simulink model "mainModelDOEJF"  (R2025a)
settings: Solver=VariableStepAuto  StartTime=0  StopTime=1000  RelTol=1e-3
undefined symbols (not defined in the file): advectiveCoefficientScale, AmbientTemperature, coolantTempSourceTemperatureScale, massCoolantScale, massModuleScale, scaledAdvectiveCoefficient, scaledCoolantTemp, scaledMassCoolant, scaledMassModule
libraries: fl_lib x265, nesl_utility x68, coolantFlow_lib x65, thermalCoupledCellResolution_lib x32, heatGenerationForCellResolvedModel x32, batt_lib x1, coolantFlowSwitch_lib x1
(part 2 of 4)

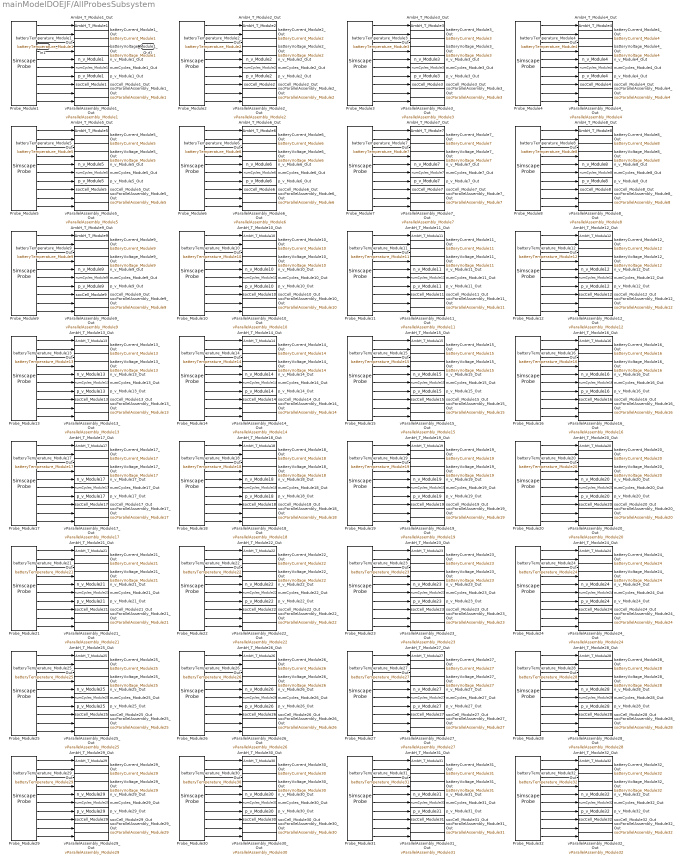
== system mainModelDOEJF/AllProbesSubsystem ==
  In1 : Inport
  AmbH_T_Module10_Out : ToWorkspace  VariableName=AmbH_T_Module10  SaveFormat=Structure With Time  SampleTime=-1
  AmbH_T_Module11_Out : ToWorkspace  VariableName=AmbH_T_Module11  SaveFormat=Structure With Time  SampleTime=-1
  AmbH_T_Module12_Out : ToWorkspace  VariableName=AmbH_T_Module12  SaveFormat=Structure With Time  SampleTime=-1
  AmbH_T_Module13_Out : ToWorkspace  VariableName=AmbH_T_Module13  SaveFormat=Structure With Time  SampleTime=-1
  AmbH_T_Module14_Out : ToWorkspace  VariableName=AmbH_T_Module14  SaveFormat=Structure With Time  SampleTime=-1
  AmbH_T_Module15_Out : ToWorkspace  VariableName=AmbH_T_Module15  SaveFormat=Structure With Time  SampleTime=-1
  AmbH_T_Module16_Out : ToWorkspace  VariableName=AmbH_T_Module16  SaveFormat=Structure With Time  SampleTime=-1
  AmbH_T_Module17_Out : ToWorkspace  VariableName=AmbH_T_Module17  SaveFormat=Structure With Time  SampleTime=-1
  AmbH_T_Module18_Out : ToWorkspace  VariableName=AmbH_T_Module18  SaveFormat=Structure With Time  SampleTime=-1
  AmbH_T_Module19_Out : ToWorkspace  VariableName=AmbH_T_Module19  SaveFormat=Structure With Time  SampleTime=-1
  AmbH_T_Module1_Out : ToWorkspace  VariableName=AmbH_T_Module1  SaveFormat=Structure With Time  SampleTime=-1
  AmbH_T_Module20_Out : ToWorkspace  VariableName=AmbH_T_Module20  SaveFormat=Structure With Time  SampleTime=-1
  AmbH_T_Module21_Out : ToWorkspace  VariableName=AmbH_T_Module21  SaveFormat=Structure With Time  SampleTime=-1
  AmbH_T_Module22_Out : ToWorkspace  VariableName=AmbH_T_Module22  SaveFormat=Structure With Time  SampleTime=-1
  AmbH_T_Module23_Out : ToWorkspace  VariableName=AmbH_T_Module23  SaveFormat=Structure With Time  SampleTime=-1
  AmbH_T_Module24_Out : ToWorkspace  VariableName=AmbH_T_Module24  SaveFormat=Structure With Time  SampleTime=-1
  AmbH_T_Module25_Out : ToWorkspace  VariableName=AmbH_T_Module25  SaveFormat=Structure With Time  SampleTime=-1
  AmbH_T_Module26_Out : ToWorkspace  VariableName=AmbH_T_Module26  SaveFormat=Structure With Time  SampleTime=-1
  AmbH_T_Module27_Out : ToWorkspace  VariableName=AmbH_T_Module27  SaveFormat=Structure With Time  SampleTime=-1
  AmbH_T_Module28_Out : ToWorkspace  VariableName=AmbH_T_Module28  SaveFormat=Structure With Time  SampleTime=-1
  AmbH_T_Module29_Out : ToWorkspace  VariableName=AmbH_T_Module29  SaveFormat=Structure With Time  SampleTime=-1
  AmbH_T_Module2_Out : ToWorkspace  VariableName=AmbH_T_Module2  SaveFormat=Structure With Time  SampleTime=-1
  AmbH_T_Module30_Out : ToWorkspace  VariableName=AmbH_T_Module30  SaveFormat=Structure With Time  SampleTime=-1
  AmbH_T_Module31_Out : ToWorkspace  VariableName=AmbH_T_Module31  SaveFormat=Structure With Time  SampleTime=-1
  AmbH_T_Module32_Out : ToWorkspace  VariableName=AmbH_T_Module32  SaveFormat=Structure With Time  SampleTime=-1
  AmbH_T_Module3_Out : ToWorkspace  VariableName=AmbH_T_Module3  SaveFormat=Structure With Time  SampleTime=-1
  AmbH_T_Module4_Out : ToWorkspace  VariableName=AmbH_T_Module4  SaveFormat=Structure With Time  SampleTime=-1
  AmbH_T_Module5_Out : ToWorkspace  VariableName=AmbH_T_Module5  SaveFormat=Structure With Time  SampleTime=-1
  AmbH_T_Module6_Out : ToWorkspace  VariableName=AmbH_T_Module6  SaveFormat=Structure With Time  SampleTime=-1
  AmbH_T_Module7_Out : ToWorkspace  VariableName=AmbH_T_Module7  SaveFormat=Structure With Time  SampleTime=-1
  AmbH_T_Module8_Out : ToWorkspace  VariableName=AmbH_T_Module8  SaveFormat=Structure With Time  SampleTime=-1
  AmbH_T_Module9_Out : ToWorkspace  VariableName=AmbH_T_Module9  SaveFormat=Structure With Time  SampleTime=-1
  Probe_Module1 : SimscapeProbe  BoundBlock=1  Variables="{\"AmbH.T\":{\"Probing\":\"ON\"},\"batteryCurrent\":{\"Probing\":\"ON\"},\"batteryTemperature\":{\"Probing\":\"ON\"},\"batteryVoltage\":{\"Probing\":\"ON\"},\"n.v\":{\"Probing\":\"ON\"},\"numCycles\":{\"Probing\":\"ON\"},\"p.v\":{\"Probing\":\"ON\"},\"socCell\":{\"Probing\":\"ON\"},\"socParallelAssembly\":{\"Probing\":\"ON\"},\"vParallelAssembly\":{\"Probing\":\"ON\"}}"
  Probe_Module10 : SimscapeProbe  BoundBlock=10  Variables="{\"AmbH.T\":{\"Probing\":\"ON\"},\"batteryCurrent\":{\"Probing\":\"ON\"},\"batteryTemperature\":{\"Probing\":\"ON\"},\"batteryVoltage\":{\"Probing\":\"ON\"},\"n.v\":{\"Probing\":\"ON\"},\"numCycles\":{\"Probing\":\"ON\"},\"p.v\":{\"Probing\":\"ON\"},\"socCell\":{\"Probing\":\"ON\"},\"socParallelAssembly\":{\"Probing\":\"ON\"},\"vParallelAssembly\":{\"Probing\":\"ON\"}}"
  Probe_Module11 : SimscapeProbe  BoundBlock=11  Variables="{\"AmbH.T\":{\"Probing\":\"ON\"},\"batteryCurrent\":{\"Probing\":\"ON\"},\"batteryTemperature\":{\"Probing\":\"ON\"},\"batteryVoltage\":{\"Probing\":\"ON\"},\"n.v\":{\"Probing\":\"ON\"},\"numCycles\":{\"Probing\":\"ON\"},\"p.v\":{\"Probing\":\"ON\"},\"socCell\":{\"Probing\":\"ON\"},\"socParallelAssembly\":{\"Probing\":\"ON\"},\"vParallelAssembly\":{\"Probing\":\"ON\"}}"
  Probe_Module12 : SimscapeProbe  BoundBlock=12  Variables="{\"AmbH.T\":{\"Probing\":\"ON\"},\"batteryCurrent\":{\"Probing\":\"ON\"},\"batteryTemperature\":{\"Probing\":\"ON\"},\"batteryVoltage\":{\"Probing\":\"ON\"},\"n.v\":{\"Probing\":\"ON\"},\"numCycles\":{\"Probing\":\"ON\"},\"p.v\":{\"Probing\":\"ON\"},\"socCell\":{\"Probing\":\"ON\"},\"socParallelAssembly\":{\"Probing\":\"ON\"},\"vParallelAssembly\":{\"Probing\":\"ON\"}}"
  Probe_Module13 : SimscapeProbe  BoundBlock=13  Variables="{\"AmbH.T\":{\"Probing\":\"ON\"},\"batteryCurrent\":{\"Probing\":\"ON\"},\"batteryTemperature\":{\"Probing\":\"ON\"},\"batteryVoltage\":{\"Probing\":\"ON\"},\"n.v\":{\"Probing\":\"ON\"},\"numCycles\":{\"Probing\":\"ON\"},\"p.v\":{\"Probing\":\"ON\"},\"socCell\":{\"Probing\":\"ON\"},\"socParallelAssembly\":{\"Probing\":\"ON\"},\"vParallelAssembly\":{\"Probing\":\"ON\"}}"
  Probe_Module14 : SimscapeProbe  BoundBlock=14  Variables="{\"AmbH.T\":{\"Probing\":\"ON\"},\"batteryCurrent\":{\"Probing\":\"ON\"},\"batteryTemperature\":{\"Probing\":\"ON\"},\"batteryVoltage\":{\"Probing\":\"ON\"},\"n.v\":{\"Probing\":\"ON\"},\"numCycles\":{\"Probing\":\"ON\"},\"p.v\":{\"Probing\":\"ON\"},\"socCell\":{\"Probing\":\"ON\"},\"socParallelAssembly\":{\"Probing\":\"ON\"},\"vParallelAssembly\":{\"Probing\":\"ON\"}}"
  Probe_Module15 : SimscapeProbe  BoundBlock=15  Variables="{\"AmbH.T\":{\"Probing\":\"ON\"},\"batteryCurrent\":{\"Probing\":\"ON\"},\"batteryTemperature\":{\"Probing\":\"ON\"},\"batteryVoltage\":{\"Probing\":\"ON\"},\"n.v\":{\"Probing\":\"ON\"},\"numCycles\":{\"Probing\":\"ON\"},\"p.v\":{\"Probing\":\"ON\"},\"socCell\":{\"Probing\":\"ON\"},\"socParallelAssembly\":{\"Probing\":\"ON\"},\"vParallelAssembly\":{\"Probing\":\"ON\"}}"
  Probe_Module16 : SimscapeProbe  BoundBlock=16  Variables="{\"AmbH.T\":{\"Probing\":\"ON\"},\"batteryCurrent\":{\"Probing\":\"ON\"},\"batteryTemperature\":{\"Probing\":\"ON\"},\"batteryVoltage\":{\"Probing\":\"ON\"},\"n.v\":{\"Probing\":\"ON\"},\"numCycles\":{\"Probing\":\"ON\"},\"p.v\":{\"Probing\":\"ON\"},\"socCell\":{\"Probing\":\"ON\"},\"socParallelAssembly\":{\"Probing\":\"ON\"},\"vParallelAssembly\":{\"Probing\":\"ON\"}}"
  Probe_Module17 : SimscapeProbe  BoundBlock=17  Variables="{\"AmbH.T\":{\"Probing\":\"ON\"},\"batteryCurrent\":{\"Probing\":\"ON\"},\"batteryTemperature\":{\"Probing\":\"ON\"},\"batteryVoltage\":{\"Probing\":\"ON\"},\"n.v\":{\"Probing\":\"ON\"},\"numCycles\":{\"Probing\":\"ON\"},\"p.v\":{\"Probing\":\"ON\"},\"socCell\":{\"Probing\":\"ON\"},\"socParallelAssembly\":{\"Probing\":\"ON\"},\"vParallelAssembly\":{\"Probing\":\"ON\"}}"
  Probe_Module18 : SimscapeProbe  BoundBlock=18  Variables="{\"AmbH.T\":{\"Probing\":\"ON\"},\"batteryCurrent\":{\"Probing\":\"ON\"},\"batteryTemperature\":{\"Probing\":\"ON\"},\"batteryVoltage\":{\"Probing\":\"ON\"},\"n.v\":{\"Probing\":\"ON\"},\"numCycles\":{\"Probing\":\"ON\"},\"p.v\":{\"Probing\":\"ON\"},\"socCell\":{\"Probing\":\"ON\"},\"socParallelAssembly\":{\"Probing\":\"ON\"},\"vParallelAssembly\":{\"Probing\":\"ON\"}}"
  Probe_Module19 : SimscapeProbe  BoundBlock=19  Variables="{\"AmbH.T\":{\"Probing\":\"ON\"},\"batteryCurrent\":{\"Probing\":\"ON\"},\"batteryTemperature\":{\"Probing\":\"ON\"},\"batteryVoltage\":{\"Probing\":\"ON\"},\"n.v\":{\"Probing\":\"ON\"},\"numCycles\":{\"Probing\":\"ON\"},\"p.v\":{\"Probing\":\"ON\"},\"socCell\":{\"Probing\":\"ON\"},\"socParallelAssembly\":{\"Probing\":\"ON\"},\"vParallelAssembly\":{\"Probing\":\"ON\"}}"
  Probe_Module2 : SimscapeProbe  BoundBlock=2  Variables="{\"AmbH.T\":{\"Probing\":\"ON\"},\"batteryCurrent\":{\"Probing\":\"ON\"},\"batteryTemperature\":{\"Probing\":\"ON\"},\"batteryVoltage\":{\"Probing\":\"ON\"},\"n.v\":{\"Probing\":\"ON\"},\"numCycles\":{\"Probing\":\"ON\"},\"p.v\":{\"Probing\":\"ON\"},\"socCell\":{\"Probing\":\"ON\"},\"socParallelAssembly\":{\"Probing\":\"ON\"},\"vParallelAssembly\":{\"Probing\":\"ON\"}}"
  Probe_Module20 : SimscapeProbe  BoundBlock=20  Variables="{\"AmbH.T\":{\"Probing\":\"ON\"},\"batteryCurrent\":{\"Probing\":\"ON\"},\"batteryTemperature\":{\"Probing\":\"ON\"},\"batteryVoltage\":{\"Probing\":\"ON\"},\"n.v\":{\"Probing\":\"ON\"},\"numCycles\":{\"Probing\":\"ON\"},\"p.v\":{\"Probing\":\"ON\"},\"socCell\":{\"Probing\":\"ON\"},\"socParallelAssembly\":{\"Probing\":\"ON\"},\"vParallelAssembly\":{\"Probing\":\"ON\"}}"
  Probe_Module21 : SimscapeProbe  BoundBlock=21  Variables="{\"AmbH.T\":{\"Probing\":\"ON\"},\"batteryCurrent\":{\"Probing\":\"ON\"},\"batteryTemperature\":{\"Probing\":\"ON\"},\"batteryVoltage\":{\"Probing\":\"ON\"},\"n.v\":{\"Probing\":\"ON\"},\"numCycles\":{\"Probing\":\"ON\"},\"p.v\":{\"Probing\":\"ON\"},\"socCell\":{\"Probing\":\"ON\"},\"socParallelAssembly\":{\"Probing\":\"ON\"},\"vParallelAssembly\":{\"Probing\":\"ON\"}}"
  Probe_Module22 : SimscapeProbe  BoundBlock=22  Variables="{\"AmbH.T\":{\"Probing\":\"ON\"},\"batteryCurrent\":{\"Probing\":\"ON\"},\"batteryTemperature\":{\"Probing\":\"ON\"},\"batteryVoltage\":{\"Probing\":\"ON\"},\"n.v\":{\"Probing\":\"ON\"},\"numCycles\":{\"Probing\":\"ON\"},\"p.v\":{\"Probing\":\"ON\"},\"socCell\":{\"Probing\":\"ON\"},\"socParallelAssembly\":{\"Probing\":\"ON\"},\"vParallelAssembly\":{\"Probing\":\"ON\"}}"
  Probe_Module23 : SimscapeProbe  BoundBlock=23  Variables="{\"AmbH.T\":{\"Probing\":\"ON\"},\"batteryCurrent\":{\"Probing\":\"ON\"},\"batteryTemperature\":{\"Probing\":\"ON\"},\"batteryVoltage\":{\"Probing\":\"ON\"},\"n.v\":{\"Probing\":\"ON\"},\"numCycles\":{\"Probing\":\"ON\"},\"p.v\":{\"Probing\":\"ON\"},\"socCell\":{\"Probing\":\"ON\"},\"socParallelAssembly\":{\"Probing\":\"ON\"},\"vParallelAssembly\":{\"Probing\":\"ON\"}}"
  Probe_Module24 : SimscapeProbe  BoundBlock=24  Variables="{\"AmbH.T\":{\"Probing\":\"ON\"},\"batteryCurrent\":{\"Probing\":\"ON\"},\"batteryTemperature\":{\"Probing\":\"ON\"},\"batteryVoltage\":{\"Probing\":\"ON\"},\"n.v\":{\"Probing\":\"ON\"},\"numCycles\":{\"Probing\":\"ON\"},\"p.v\":{\"Probing\":\"ON\"},\"socCell\":{\"Probing\":\"ON\"},\"socParallelAssembly\":{\"Probing\":\"ON\"},\"vParallelAssembly\":{\"Probing\":\"ON\"}}"
  Probe_Module25 : SimscapeProbe  BoundBlock=25  Variables="{\"AmbH.T\":{\"Probing\":\"ON\"},\"batteryCurrent\":{\"Probing\":\"ON\"},\"batteryTemperature\":{\"Probing\":\"ON\"},\"batteryVoltage\":{\"Probing\":\"ON\"},\"n.v\":{\"Probing\":\"ON\"},\"numCycles\":{\"Probing\":\"ON\"},\"p.v\":{\"Probing\":\"ON\"},\"socCell\":{\"Probing\":\"ON\"},\"socParallelAssembly\":{\"Probing\":\"ON\"},\"vParallelAssembly\":{\"Probing\":\"ON\"}}"
  Probe_Module26 : SimscapeProbe  BoundBlock=26  Variables="{\"AmbH.T\":{\"Probing\":\"ON\"},\"batteryCurrent\":{\"Probing\":\"ON\"},\"batteryTemperature\":{\"Probing\":\"ON\"},\"batteryVoltage\":{\"Probing\":\"ON\"},\"n.v\":{\"Probing\":\"ON\"},\"numCycles\":{\"Probing\":\"ON\"},\"p.v\":{\"Probing\":\"ON\"},\"socCell\":{\"Probing\":\"ON\"},\"socParallelAssembly\":{\"Probing\":\"ON\"},\"vParallelAssembly\":{\"Probing\":\"ON\"}}"
  Probe_Module27 : SimscapeProbe  BoundBlock=27  Variables="{\"AmbH.T\":{\"Probing\":\"ON\"},\"batteryCurrent\":{\"Probing\":\"ON\"},\"batteryTemperature\":{\"Probing\":\"ON\"},\"batteryVoltage\":{\"Probing\":\"ON\"},\"n.v\":{\"Probing\":\"ON\"},\"numCycles\":{\"Probing\":\"ON\"},\"p.v\":{\"Probing\":\"ON\"},\"socCell\":{\"Probing\":\"ON\"},\"socParallelAssembly\":{\"Probing\":\"ON\"},\"vParallelAssembly\":{\"Probing\":\"ON\"}}"
  Probe_Module28 : SimscapeProbe  BoundBlock=28  Variables="{\"AmbH.T\":{\"Probing\":\"ON\"},\"batteryCurrent\":{\"Probing\":\"ON\"},\"batteryTemperature\":{\"Probing\":\"ON\"},\"batteryVoltage\":{\"Probing\":\"ON\"},\"n.v\":{\"Probing\":\"ON\"},\"numCycles\":{\"Probing\":\"ON\"},\"p.v\":{\"Probing\":\"ON\"},\"socCell\":{\"Probing\":\"ON\"},\"socParallelAssembly\":{\"Probing\":\"ON\"},\"vParallelAssembly\":{\"Probing\":\"ON\"}}"
  Probe_Module29 : SimscapeProbe  BoundBlock=29  Variables="{\"AmbH.T\":{\"Probing\":\"ON\"},\"batteryCurrent\":{\"Probing\":\"ON\"},\"batteryTemperature\":{\"Probing\":\"ON\"},\"batteryVoltage\":{\"Probing\":\"ON\"},\"n.v\":{\"Probing\":\"ON\"},\"numCycles\":{\"Probing\":\"ON\"},\"p.v\":{\"Probing\":\"ON\"},\"socCell\":{\"Probing\":\"ON\"},\"socParallelAssembly\":{\"Probing\":\"ON\"},\"vParallelAssembly\":{\"Probing\":\"ON\"}}"
  Probe_Module3 : SimscapeProbe  BoundBlock=3  Variables="{\"AmbH.T\":{\"Probing\":\"ON\"},\"batteryCurrent\":{\"Probing\":\"ON\"},\"batteryTemperature\":{\"Probing\":\"ON\"},\"batteryVoltage\":{\"Probing\":\"ON\"},\"n.v\":{\"Probing\":\"ON\"},\"numCycles\":{\"Probing\":\"ON\"},\"p.v\":{\"Probing\":\"ON\"},\"socCell\":{\"Probing\":\"ON\"},\"socParallelAssembly\":{\"Probing\":\"ON\"},\"vParallelAssembly\":{\"Probing\":\"ON\"}}"
  Probe_Module30 : SimscapeProbe  BoundBlock=30  Variables="{\"AmbH.T\":{\"Probing\":\"ON\"},\"batteryCurrent\":{\"Probing\":\"ON\"},\"batteryTemperature\":{\"Probing\":\"ON\"},\"batteryVoltage\":{\"Probing\":\"ON\"},\"n.v\":{\"Probing\":\"ON\"},\"numCycles\":{\"Probing\":\"ON\"},\"p.v\":{\"Probing\":\"ON\"},\"socCell\":{\"Probing\":\"ON\"},\"socParallelAssembly\":{\"Probing\":\"ON\"},\"vParallelAssembly\":{\"Probing\":\"ON\"}}"
  Probe_Module31 : SimscapeProbe  BoundBlock=31  Variables="{\"AmbH.T\":{\"Probing\":\"ON\"},\"batteryCurrent\":{\"Probing\":\"ON\"},\"batteryTemperature\":{\"Probing\":\"ON\"},\"batteryVoltage\":{\"Probing\":\"ON\"},\"n.v\":{\"Probing\":\"ON\"},\"numCycles\":{\"Probing\":\"ON\"},\"p.v\":{\"Probing\":\"ON\"},\"socCell\":{\"Probing\":\"ON\"},\"socParallelAssembly\":{\"Probing\":\"ON\"},\"vParallelAssembly\":{\"Probing\":\"ON\"}}"
  Probe_Module32 : SimscapeProbe  BoundBlock=32  Variables="{\"AmbH.T\":{\"Probing\":\"ON\"},\"batteryCurrent\":{\"Probing\":\"ON\"},\"batteryTemperature\":{\"Probing\":\"ON\"},\"batteryVoltage\":{\"Probing\":\"ON\"},\"n.v\":{\"Probing\":\"ON\"},\"numCycles\":{\"Probing\":\"ON\"},\"p.v\":{\"Probing\":\"ON\"},\"socCell\":{\"Probing\":\"ON\"},\"socParallelAssembly\":{\"Probing\":\"ON\"},\"vParallelAssembly\":{\"Probing\":\"ON\"}}"
  Probe_Module4 : SimscapeProbe  BoundBlock=4  Variables="{\"AmbH.T\":{\"Probing\":\"ON\"},\"batteryCurrent\":{\"Probing\":\"ON\"},\"batteryTemperature\":{\"Probing\":\"ON\"},\"batteryVoltage\":{\"Probing\":\"ON\"},\"n.v\":{\"Probing\":\"ON\"},\"numCycles\":{\"Probing\":\"ON\"},\"p.v\":{\"Probing\":\"ON\"},\"socCell\":{\"Probing\":\"ON\"},\"socParallelAssembly\":{\"Probing\":\"ON\"},\"vParallelAssembly\":{\"Probing\":\"ON\"}}"
  Probe_Module5 : SimscapeProbe  BoundBlock=5  Variables="{\"AmbH.T\":{\"Probing\":\"ON\"},\"batteryCurrent\":{\"Probing\":\"ON\"},\"batteryTemperature\":{\"Probing\":\"ON\"},\"batteryVoltage\":{\"Probing\":\"ON\"},\"n.v\":{\"Probing\":\"ON\"},\"numCycles\":{\"Probing\":\"ON\"},\"p.v\":{\"Probing\":\"ON\"},\"socCell\":{\"Probing\":\"ON\"},\"socParallelAssembly\":{\"Probing\":\"ON\"},\"vParallelAssembly\":{\"Probing\":\"ON\"}}"
  Probe_Module6 : SimscapeProbe  BoundBlock=6  Variables="{\"AmbH.T\":{\"Probing\":\"ON\"},\"batteryCurrent\":{\"Probing\":\"ON\"},\"batteryTemperature\":{\"Probing\":\"ON\"},\"batteryVoltage\":{\"Probing\":\"ON\"},\"n.v\":{\"Probing\":\"ON\"},\"numCycles\":{\"Probing\":\"ON\"},\"p.v\":{\"Probing\":\"ON\"},\"socCell\":{\"Probing\":\"ON\"},\"socParallelAssembly\":{\"Probing\":\"ON\"},\"vParallelAssembly\":{\"Probing\":\"ON\"}}"
  Probe_Module7 : SimscapeProbe  BoundBlock=7  Variables="{\"AmbH.T\":{\"Probing\":\"ON\"},\"batteryCurrent\":{\"Probing\":\"ON\"},\"batteryTemperature\":{\"Probing\":\"ON\"},\"batteryVoltage\":{\"Probing\":\"ON\"},\"n.v\":{\"Probing\":\"ON\"},\"numCycles\":{\"Probing\":\"ON\"},\"p.v\":{\"Probing\":\"ON\"},\"socCell\":{\"Probing\":\"ON\"},\"socParallelAssembly\":{\"Probing\":\"ON\"},\"vParallelAssembly\":{\"Probing\":\"ON\"}}"
  Probe_Module8 : SimscapeProbe  BoundBlock=8  Variables="{\"AmbH.T\":{\"Probing\":\"ON\"},\"batteryCurrent\":{\"Probing\":\"ON\"},\"batteryTemperature\":{\"Probing\":\"ON\"},\"batteryVoltage\":{\"Probing\":\"ON\"},\"n.v\":{\"Probing\":\"ON\"},\"numCycles\":{\"Probing\":\"ON\"},\"p.v\":{\"Probing\":\"ON\"},\"socCell\":{\"Probing\":\"ON\"},\"socParallelAssembly\":{\"Probing\":\"ON\"},\"vParallelAssembly\":{\"Probing\":\"ON\"}}"
  Probe_Module9 : SimscapeProbe  BoundBlock=9  Variables="{\"AmbH.T\":{\"Probing\":\"ON\"},\"batteryCurrent\":{\"Probing\":\"ON\"},\"batteryTemperature\":{\"Probing\":\"ON\"},\"batteryVoltage\":{\"Probing\":\"ON\"},\"n.v\":{\"Probing\":\"ON\"},\"numCycles\":{\"Probing\":\"ON\"},\"p.v\":{\"Probing\":\"ON\"},\"socCell\":{\"Probing\":\"ON\"},\"socParallelAssembly\":{\"Probing\":\"ON\"},\"vParallelAssembly\":{\"Probing\":\"ON\"}}"
  batteryCurrent_Module10_Out : ToWorkspace  VariableName=batteryCurrent_Module10  SaveFormat=Structure With Time  SampleTime=-1
  batteryCurrent_Module11_Out : ToWorkspace  VariableName=batteryCurrent_Module11  SaveFormat=Structure With Time  SampleTime=-1
  batteryCurrent_Module12_Out : ToWorkspace  VariableName=batteryCurrent_Module12  SaveFormat=Structure With Time  SampleTime=-1
  batteryCurrent_Module13_Out : ToWorkspace  VariableName=batteryCurrent_Module13  SaveFormat=Structure With Time  SampleTime=-1
  batteryCurrent_Module14_Out : ToWorkspace  VariableName=batteryCurrent_Module14  SaveFormat=Structure With Time  SampleTime=-1
  batteryCurrent_Module15_Out : ToWorkspace  VariableName=batteryCurrent_Module15  SaveFormat=Structure With Time  SampleTime=-1
  batteryCurrent_Module16_Out : ToWorkspace  VariableName=batteryCurrent_Module16  SaveFormat=Structure With Time  SampleTime=-1
  batteryCurrent_Module17_Out : ToWorkspace  VariableName=batteryCurrent_Module17  SaveFormat=Structure With Time  SampleTime=-1
  batteryCurrent_Module18_Out : ToWorkspace  VariableName=batteryCurrent_Module18  SaveFormat=Structure With Time  SampleTime=-1
  batteryCurrent_Module19_Out : ToWorkspace  VariableName=batteryCurrent_Module19  SaveFormat=Structure With Time  SampleTime=-1
  batteryCurrent_Module1_Out : ToWorkspace  VariableName=batteryCurrent_Module1  SaveFormat=Structure With Time  SampleTime=-1
  batteryCurrent_Module20_Out : ToWorkspace  VariableName=batteryCurrent_Module20  SaveFormat=Structure With Time  SampleTime=-1
  batteryCurrent_Module21_Out : ToWorkspace  VariableName=batteryCurrent_Module21  SaveFormat=Structure With Time  SampleTime=-1
  batteryCurrent_Module22_Out : ToWorkspace  VariableName=batteryCurrent_Module22  SaveFormat=Structure With Time  SampleTime=-1
  batteryCurrent_Module23_Out : ToWorkspace  VariableName=batteryCurrent_Module23  SaveFormat=Structure With Time  SampleTime=-1
  batteryCurrent_Module24_Out : ToWorkspace  VariableName=batteryCurrent_Module24  SaveFormat=Structure With Time  SampleTime=-1
  batteryCurrent_Module25_Out : ToWorkspace  VariableName=batteryCurrent_Module25  SaveFormat=Structure With Time  SampleTime=-1
  batteryCurrent_Module26_Out : ToWorkspace  VariableName=batteryCurrent_Module26  SaveFormat=Structure With Time  SampleTime=-1
  batteryCurrent_Module27_Out : ToWorkspace  VariableName=batteryCurrent_Module27  SaveFormat=Structure With Time  SampleTime=-1
  batteryCurrent_Module28_Out : ToWorkspace  VariableName=batteryCurrent_Module28  SaveFormat=Structure With Time  SampleTime=-1
  batteryCurrent_Module29_Out : ToWorkspace  VariableName=batteryCurrent_Module29  SaveFormat=Structure With Time  SampleTime=-1
  batteryCurrent_Module2_Out : ToWorkspace  VariableName=batteryCurrent_Module2  SaveFormat=Structure With Time  SampleTime=-1
  batteryCurrent_Module30_Out : ToWorkspace  VariableName=batteryCurrent_Module30  SaveFormat=Structure With Time  SampleTime=-1
  batteryCurrent_Module31_Out : ToWorkspace  VariableName=batteryCurrent_Module31  SaveFormat=Structure With Time  SampleTime=-1
  batteryCurrent_Module32_Out : ToWorkspace  VariableName=batteryCurrent_Module32  SaveFormat=Structure With Time  SampleTime=-1
  batteryCurrent_Module3_Out : ToWorkspace  VariableName=batteryCurrent_Module3  SaveFormat=Structure With Time  SampleTime=-1
  batteryCurrent_Module4_Out : ToWorkspace  VariableName=batteryCurrent_Module4  SaveFormat=Structure With Time  SampleTime=-1
  batteryCurrent_Module5_Out : ToWorkspace  VariableName=batteryCurrent_Module5  SaveFormat=Structure With Time  SampleTime=-1
  batteryCurrent_Module6_Out : ToWorkspace  VariableName=batteryCurrent_Module6  SaveFormat=Structure With Time  SampleTime=-1
  batteryCurrent_Module7_Out : ToWorkspace  VariableName=batteryCurrent_Module7  SaveFormat=Structure With Time  SampleTime=-1
  batteryCurrent_Module8_Out : ToWorkspace  VariableName=batteryCurrent_Module8  SaveFormat=Structure With Time  SampleTime=-1
  batteryCurrent_Module9_Out : ToWorkspace  VariableName=batteryCurrent_Module9  SaveFormat=Structure With Time  SampleTime=-1
  batteryTemperature_Module10_Out : ToWorkspace  VariableName=batteryTemperature_Module10  SaveFormat=Structure With Time  SampleTime=-1
  batteryTemperature_Module11_Out : ToWorkspace  VariableName=batteryTemperature_Module11  SaveFormat=Structure With Time  SampleTime=-1
  batteryTemperature_Module12_Out : ToWorkspace  VariableName=batteryTemperature_Module12  SaveFormat=Structure With Time  SampleTime=-1
  batteryTemperature_Module13_Out : ToWorkspace  VariableName=batteryTemperature_Module13  SaveFormat=Structure With Time  SampleTime=-1
  batteryTemperature_Module14_Out : ToWorkspace  VariableName=batteryTemperature_Module14  SaveFormat=Structure With Time  SampleTime=-1
  batteryTemperature_Module15_Out : ToWorkspace  VariableName=batteryTemperature_Module15  SaveFormat=Structure With Time  SampleTime=-1
  batteryTemperature_Module16_Out : ToWorkspace  VariableName=batteryTemperature_Module16  SaveFormat=Structure With Time  SampleTime=-1
  batteryTemperature_Module17_Out : ToWorkspace  VariableName=batteryTemperature_Module17  SaveFormat=Structure With Time  SampleTime=-1
  batteryTemperature_Module18_Out : ToWorkspace  VariableName=batteryTemperature_Module18  SaveFormat=Structure With Time  SampleTime=-1
  batteryTemperature_Module19_Out : ToWorkspace  VariableName=batteryTemperature_Module19  SaveFormat=Structure With Time  SampleTime=-1
  batteryTemperature_Module1_Out : ToWorkspace  VariableName=batteryTemperature_Module1  SaveFormat=Structure With Time  SampleTime=-1
  batteryTemperature_Module20_Out : ToWorkspace  VariableName=batteryTemperature_Module20  SaveFormat=Structure With Time  SampleTime=-1
  batteryTemperature_Module21_Out : ToWorkspace  VariableName=batteryTemperature_Module21  SaveFormat=Structure With Time  SampleTime=-1
  batteryTemperature_Module22_Out : ToWorkspace  VariableName=batteryTemperature_Module22  SaveFormat=Structure With Time  SampleTime=-1
  batteryTemperature_Module23_Out : ToWorkspace  VariableName=batteryTemperature_Module23  SaveFormat=Structure With Time  SampleTime=-1
  batteryTemperature_Module24_Out : ToWorkspace  VariableName=batteryTemperature_Module24  SaveFormat=Structure With Time  SampleTime=-1
  batteryTemperature_Module25_Out : ToWorkspace  VariableName=batteryTemperature_Module25  SaveFormat=Structure With Time  SampleTime=-1
  batteryTemperature_Module26_Out : ToWorkspace  VariableName=batteryTemperature_Module26  SaveFormat=Structure With Time  SampleTime=-1
  batteryTemperature_Module27_Out : ToWorkspace  VariableName=batteryTemperature_Module27  SaveFormat=Structure With Time  SampleTime=-1
  batteryTemperature_Module28_Out : ToWorkspace  VariableName=batteryTemperature_Module28  SaveFormat=Structure With Time  SampleTime=-1
  batteryTemperature_Module29_Out : ToWorkspace  VariableName=batteryTemperature_Module29  SaveFormat=Structure With Time  SampleTime=-1
  batteryTemperature_Module2_Out : ToWorkspace  VariableName=batteryTemperature_Module2  SaveFormat=Structure With Time  SampleTime=-1
  batteryTemperature_Module30_Out : ToWorkspace  VariableName=batteryTemperature_Module30  SaveFormat=Structure With Time  SampleTime=-1
  batteryTemperature_Module31_Out : ToWorkspace  VariableName=batteryTemperature_Module31  SaveFormat=Structure With Time  SampleTime=-1
  batteryTemperature_Module32_Out : ToWorkspace  VariableName=batteryTemperature_Module32  SaveFormat=Structure With Time  SampleTime=-1
  batteryTemperature_Module3_Out : ToWorkspace  VariableName=batteryTemperature_Module3  SaveFormat=Structure With Time  SampleTime=-1
  batteryTemperature_Module4_Out : ToWorkspace  VariableName=batteryTemperature_Module4  SaveFormat=Structure With Time  SampleTime=-1
  batteryTemperature_Module5_Out : ToWorkspace  VariableName=batteryTemperature_Module5  SaveFormat=Structure With Time  SampleTime=-1
  batteryTemperature_Module6_Out : ToWorkspace  VariableName=batteryTemperature_Module6  SaveFormat=Structure With Time  SampleTime=-1
  batteryTemperature_Module7_Out : ToWorkspace  VariableName=batteryTemperature_Module7  SaveFormat=Structure With Time  SampleTime=-1
  batteryTemperature_Module8_Out : ToWorkspace  VariableName=batteryTemperature_Module8  SaveFormat=Structure With Time  SampleTime=-1
  batteryTemperature_Module9_Out : ToWorkspace  VariableName=batteryTemperature_Module9  SaveFormat=Structure With Time  SampleTime=-1
  batteryVoltage_Module10_Out : ToWorkspace  VariableName=batteryVoltage_Module10  SaveFormat=Structure With Time  SampleTime=-1
  batteryVoltage_Module11_Out : ToWorkspace  VariableName=batteryVoltage_Module11  SaveFormat=Structure With Time  SampleTime=-1
  batteryVoltage_Module12_Out : ToWorkspace  VariableName=batteryVoltage_Module12  SaveFormat=Structure With Time  SampleTime=-1
  batteryVoltage_Module13_Out : ToWorkspace  VariableName=batteryVoltage_Module13  SaveFormat=Structure With Time  SampleTime=-1
  batteryVoltage_Module14_Out : ToWorkspace  VariableName=batteryVoltage_Module14  SaveFormat=Structure With Time  SampleTime=-1
  batteryVoltage_Module15_Out : ToWorkspace  VariableName=batteryVoltage_Module15  SaveFormat=Structure With Time  SampleTime=-1
  batteryVoltage_Module16_Out : ToWorkspace  VariableName=batteryVoltage_Module16  SaveFormat=Structure With Time  SampleTime=-1
  batteryVoltage_Module17_Out : ToWorkspace  VariableName=batteryVoltage_Module17  SaveFormat=Structure With Time  SampleTime=-1
  batteryVoltage_Module18_Out : ToWorkspace  VariableName=batteryVoltage_Module18  SaveFormat=Structure With Time  SampleTime=-1
  batteryVoltage_Module19_Out : ToWorkspace  VariableName=batteryVoltage_Module19  SaveFormat=Structure With Time  SampleTime=-1
  batteryVoltage_Module1_Out : ToWorkspace  VariableName=batteryVoltage_Module1  SaveFormat=Structure With Time  SampleTime=-1
  batteryVoltage_Module20_Out : ToWorkspace  VariableName=batteryVoltage_Module20  SaveFormat=Structure With Time  SampleTime=-1
  batteryVoltage_Module21_Out : ToWorkspace  VariableName=batteryVoltage_Module21  SaveFormat=Structure With Time  SampleTime=-1
  batteryVoltage_Module22_Out : ToWorkspace  VariableName=batteryVoltage_Module22  SaveFormat=Structure With Time  SampleTime=-1
  batteryVoltage_Module23_Out : ToWorkspace  VariableName=batteryVoltage_Module23  SaveFormat=Structure With Time  SampleTime=-1
  batteryVoltage_Module24_Out : ToWorkspace  VariableName=batteryVoltage_Module24  SaveFormat=Structure With Time  SampleTime=-1
  batteryVoltage_Module25_Out : ToWorkspace  VariableName=batteryVoltage_Module25  SaveFormat=Structure With Time  SampleTime=-1
  batteryVoltage_Module26_Out : ToWorkspace  VariableName=batteryVoltage_Module26  SaveFormat=Structure With Time  SampleTime=-1
  batteryVoltage_Module27_Out : ToWorkspace  VariableName=batteryVoltage_Module27  SaveFormat=Structure With Time  SampleTime=-1
  batteryVoltage_Module28_Out : ToWorkspace  VariableName=batteryVoltage_Module28  SaveFormat=Structure With Time  SampleTime=-1
  batteryVoltage_Module29_Out : ToWorkspace  VariableName=batteryVoltage_Module29  SaveFormat=Structure With Time  SampleTime=-1
  batteryVoltage_Module2_Out : ToWorkspace  VariableName=batteryVoltage_Module2  SaveFormat=Structure With Time  SampleTime=-1
  batteryVoltage_Module30_Out : ToWorkspace  VariableName=batteryVoltage_Module30  SaveFormat=Structure With Time  SampleTime=-1
  batteryVoltage_Module31_Out : ToWorkspace  VariableName=batteryVoltage_Module31  SaveFormat=Structure With Time  SampleTime=-1
  batteryVoltage_Module32_Out : ToWorkspace  VariableName=batteryVoltage_Module32  SaveFormat=Structure With Time  SampleTime=-1
  batteryVoltage_Module3_Out : ToWorkspace  VariableName=batteryVoltage_Module3  SaveFormat=Structure With Time  SampleTime=-1
  batteryVoltage_Module4_Out : ToWorkspace  VariableName=batteryVoltage_Module4  SaveFormat=Structure With Time  SampleTime=-1
  batteryVoltage_Module5_Out : ToWorkspace  VariableName=batteryVoltage_Module5  SaveFormat=Structure With Time  SampleTime=-1
  batteryVoltage_Module6_Out : ToWorkspace  VariableName=batteryVoltage_Module6  SaveFormat=Structure With Time  SampleTime=-1
  batteryVoltage_Module7_Out : ToWorkspace  VariableName=batteryVoltage_Module7  SaveFormat=Structure With Time  SampleTime=-1
  batteryVoltage_Module8_Out : ToWorkspace  VariableName=batteryVoltage_Module8  SaveFormat=Structure With Time  SampleTime=-1
  batteryVoltage_Module9_Out : ToWorkspace  VariableName=batteryVoltage_Module9  SaveFormat=Structure With Time  SampleTime=-1
  n_v_Module10_Out : ToWorkspace  VariableName=n_v_Module10  SaveFormat=Structure With Time  SampleTime=-1
  n_v_Module11_Out : ToWorkspace  VariableName=n_v_Module11  SaveFormat=Structure With Time  SampleTime=-1
  n_v_Module12_Out : ToWorkspace  VariableName=n_v_Module12  SaveFormat=Structure With Time  SampleTime=-1
  n_v_Module13_Out : ToWorkspace  VariableName=n_v_Module13  SaveFormat=Structure With Time  SampleTime=-1
  n_v_Module14_Out : ToWorkspace  VariableName=n_v_Module14  SaveFormat=Structure With Time  SampleTime=-1
  n_v_Module15_Out : ToWorkspace  VariableName=n_v_Module15  SaveFormat=Structure With Time  SampleTime=-1
  n_v_Module16_Out : ToWorkspace  VariableName=n_v_Module16  SaveFormat=Structure With Time  SampleTime=-1
  n_v_Module17_Out : ToWorkspace  VariableName=n_v_Module17  SaveFormat=Structure With Time  SampleTime=-1
  n_v_Module18_Out : ToWorkspace  VariableName=n_v_Module18  SaveFormat=Structure With Time  SampleTime=-1
  n_v_Module19_Out : ToWorkspace  VariableName=n_v_Module19  SaveFormat=Structure With Time  SampleTime=-1
  n_v_Module1_Out : ToWorkspace  VariableName=n_v_Module1  SaveFormat=Structure With Time  SampleTime=-1
  n_v_Module20_Out : ToWorkspace  VariableName=n_v_Module20  SaveFormat=Structure With Time  SampleTime=-1
  n_v_Module21_Out : ToWorkspace  VariableName=n_v_Module21  SaveFormat=Structure With Time  SampleTime=-1
  n_v_Module22_Out : ToWorkspace  VariableName=n_v_Module22  SaveFormat=Structure With Time  SampleTime=-1
  n_v_Module23_Out : ToWorkspace  VariableName=n_v_Module23  SaveFormat=Structure With Time  SampleTime=-1
  n_v_Module24_Out : ToWorkspace  VariableName=n_v_Module24  SaveFormat=Structure With Time  SampleTime=-1
  n_v_Module25_Out : ToWorkspace  VariableName=n_v_Module25  SaveFormat=Structure With Time  SampleTime=-1
  n_v_Module26_Out : ToWorkspace  VariableName=n_v_Module26  SaveFormat=Structure With Time  SampleTime=-1
  n_v_Module27_Out : ToWorkspace  VariableName=n_v_Module27  SaveFormat=Structure With Time  SampleTime=-1
  n_v_Module28_Out : ToWorkspace  VariableName=n_v_Module28  SaveFormat=Structure With Time  SampleTime=-1
  n_v_Module29_Out : ToWorkspace  VariableName=n_v_Module29  SaveFormat=Structure With Time  SampleTime=-1
  n_v_Module2_Out : ToWorkspace  VariableName=n_v_Module2  SaveFormat=Structure With Time  SampleTime=-1
  n_v_Module30_Out : ToWorkspace  VariableName=n_v_Module30  SaveFormat=Structure With Time  SampleTime=-1
  n_v_Module31_Out : ToWorkspace  VariableName=n_v_Module31  SaveFormat=Structure With Time  SampleTime=-1
  n_v_Module32_Out : ToWorkspace  VariableName=n_v_Module32  SaveFormat=Structure With Time  SampleTime=-1
  n_v_Module3_Out : ToWorkspace  VariableName=n_v_Module3  SaveFormat=Structure With Time  SampleTime=-1
  n_v_Module4_Out : ToWorkspace  VariableName=n_v_Module4  SaveFormat=Structure With Time  SampleTime=-1
  n_v_Module5_Out : ToWorkspace  VariableName=n_v_Module5  SaveFormat=Structure With Time  SampleTime=-1
  n_v_Module6_Out : ToWorkspace  VariableName=n_v_Module6  SaveFormat=Structure With Time  SampleTime=-1
  n_v_Module7_Out : ToWorkspace  VariableName=n_v_Module7  SaveFormat=Structure With Time  SampleTime=-1
  n_v_Module8_Out : ToWorkspace  VariableName=n_v_Module8  SaveFormat=Structure With Time  SampleTime=-1
  n_v_Module9_Out : ToWorkspace  VariableName=n_v_Module9  SaveFormat=Structure With Time  SampleTime=-1
  numCycles_Module10_Out : ToWorkspace  VariableName=numCycles_Module10  SaveFormat=Structure With Time  SampleTime=-1
  numCycles_Module11_Out : ToWorkspace  VariableName=numCycles_Module11  SaveFormat=Structure With Time  SampleTime=-1
  numCycles_Module12_Out : ToWorkspace  VariableName=numCycles_Module12  SaveFormat=Structure With Time  SampleTime=-1
  numCycles_Module13_Out : ToWorkspace  VariableName=numCycles_Module13  SaveFormat=Structure With Time  SampleTime=-1
  numCycles_Module14_Out : ToWorkspace  VariableName=numCycles_Module14  SaveFormat=Structure With Time  SampleTime=-1
  numCycles_Module15_Out : ToWorkspace  VariableName=numCycles_Module15  SaveFormat=Structure With Time  SampleTime=-1
  numCycles_Module16_Out : ToWorkspace  VariableName=numCycles_Module16  SaveFormat=Structure With Time  SampleTime=-1
  numCycles_Module17_Out : ToWorkspace  VariableName=numCycles_Module17  SaveFormat=Structure With Time  SampleTime=-1
  numCycles_Module18_Out : ToWorkspace  VariableName=numCycles_Module18  SaveFormat=Structure With Time  SampleTime=-1
  numCycles_Module19_Out : ToWorkspace  VariableName=numCycles_Module19  SaveFormat=Structure With Time  SampleTime=-1
  numCycles_Module1_Out : ToWorkspace  VariableName=numCycles_Module1  SaveFormat=Structure With Time  SampleTime=-1
  numCycles_Module20_Out : ToWorkspace  VariableName=numCycles_Module20  SaveFormat=Structure With Time  SampleTime=-1
  numCycles_Module21_Out : ToWorkspace  VariableName=numCycles_Module21  SaveFormat=Structure With Time  SampleTime=-1
  numCycles_Module22_Out : ToWorkspace  VariableName=numCycles_Module22  SaveFormat=Structure With Time  SampleTime=-1
  numCycles_Module23_Out : ToWorkspace  VariableName=numCycles_Module23  SaveFormat=Structure With Time  SampleTime=-1
  numCycles_Module24_Out : ToWorkspace  VariableName=numCycles_Module24  SaveFormat=Structure With Time  SampleTime=-1
  numCycles_Module25_Out : ToWorkspace  VariableName=numCycles_Module25  SaveFormat=Structure With Time  SampleTime=-1
  numCycles_Module26_Out : ToWorkspace  VariableName=numCycles_Module26  SaveFormat=Structure With Time  SampleTime=-1
  numCycles_Module27_Out : ToWorkspace  VariableName=numCycles_Module27  SaveFormat=Structure With Time  SampleTime=-1
  numCycles_Module28_Out : ToWorkspace  VariableName=numCycles_Module28  SaveFormat=Structure With Time  SampleTime=-1
  numCycles_Module29_Out : ToWorkspace  VariableName=numCycles_Module29  SaveFormat=Structure With Time  SampleTime=-1
  numCycles_Module2_Out : ToWorkspace  VariableName=numCycles_Module2  SaveFormat=Structure With Time  SampleTime=-1
  numCycles_Module30_Out : ToWorkspace  VariableName=numCycles_Module30  SaveFormat=Structure With Time  SampleTime=-1
  numCycles_Module31_Out : ToWorkspace  VariableName=numCycles_Module31  SaveFormat=Structure With Time  SampleTime=-1
  numCycles_Module32_Out : ToWorkspace  VariableName=numCycles_Module32  SaveFormat=Structure With Time  SampleTime=-1
  numCycles_Module3_Out : ToWorkspace  VariableName=numCycles_Module3  SaveFormat=Structure With Time  SampleTime=-1
  numCycles_Module4_Out : ToWorkspace  VariableName=numCycles_Module4  SaveFormat=Structure With Time  SampleTime=-1
  numCycles_Module5_Out : ToWorkspace  VariableName=numCycles_Module5  SaveFormat=Structure With Time  SampleTime=-1
  numCycles_Module6_Out : ToWorkspace  VariableName=numCycles_Module6  SaveFormat=Structure With Time  SampleTime=-1
  numCycles_Module7_Out : ToWorkspace  VariableName=numCycles_Module7  SaveFormat=Structure With Time  SampleTime=-1
  numCycles_Module8_Out : ToWorkspace  VariableName=numCycles_Module8  SaveFormat=Structure With Time  SampleTime=-1
  numCycles_Module9_Out : ToWorkspace  VariableName=numCycles_Module9  SaveFormat=Structure With Time  SampleTime=-1
  p_v_Module10_Out : ToWorkspace  VariableName=p_v_Module10  SaveFormat=Structure With Time  SampleTime=-1
  p_v_Module11_Out : ToWorkspace  VariableName=p_v_Module11  SaveFormat=Structure With Time  SampleTime=-1
  p_v_Module12_Out : ToWorkspace  VariableName=p_v_Module12  SaveFormat=Structure With Time  SampleTime=-1
  p_v_Module13_Out : ToWorkspace  VariableName=p_v_Module13  SaveFormat=Structure With Time  SampleTime=-1
  p_v_Module14_Out : ToWorkspace  VariableName=p_v_Module14  SaveFormat=Structure With Time  SampleTime=-1
  p_v_Module15_Out : ToWorkspace  VariableName=p_v_Module15  SaveFormat=Structure With Time  SampleTime=-1
  p_v_Module16_Out : ToWorkspace  VariableName=p_v_Module16  SaveFormat=Structure With Time  SampleTime=-1
  p_v_Module17_Out : ToWorkspace  VariableName=p_v_Module17  SaveFormat=Structure With Time  SampleTime=-1
  p_v_Module18_Out : ToWorkspace  VariableName=p_v_Module18  SaveFormat=Structure With Time  SampleTime=-1
  p_v_Module19_Out : ToWorkspace  VariableName=p_v_Module19  SaveFormat=Structure With Time  SampleTime=-1
  p_v_Module1_Out : ToWorkspace  VariableName=p_v_Module1  SaveFormat=Structure With Time  SampleTime=-1
  p_v_Module20_Out : ToWorkspace  VariableName=p_v_Module20  SaveFormat=Structure With Time  SampleTime=-1
  p_v_Module21_Out : ToWorkspace  VariableName=p_v_Module21  SaveFormat=Structure With Time  SampleTime=-1
  p_v_Module22_Out : ToWorkspace  VariableName=p_v_Module22  SaveFormat=Structure With Time  SampleTime=-1
  p_v_Module23_Out : ToWorkspace  VariableName=p_v_Module23  SaveFormat=Structure With Time  SampleTime=-1
  p_v_Module24_Out : ToWorkspace  VariableName=p_v_Module24  SaveFormat=Structure With Time  SampleTime=-1
  p_v_Module25_Out : ToWorkspace  VariableName=p_v_Module25  SaveFormat=Structure With Time  SampleTime=-1
  p_v_Module26_Out : ToWorkspace  VariableName=p_v_Module26  SaveFormat=Structure With Time  SampleTime=-1
  p_v_Module27_Out : ToWorkspace  VariableName=p_v_Module27  SaveFormat=Structure With Time  SampleTime=-1
  p_v_Module28_Out : ToWorkspace  VariableName=p_v_Module28  SaveFormat=Structure With Time  SampleTime=-1
  p_v_Module29_Out : ToWorkspace  VariableName=p_v_Module29  SaveFormat=Structure With Time  SampleTime=-1
  p_v_Module2_Out : ToWorkspace  VariableName=p_v_Module2  SaveFormat=Structure With Time  SampleTime=-1
  p_v_Module30_Out : ToWorkspace  VariableName=p_v_Module30  SaveFormat=Structure With Time  SampleTime=-1
  p_v_Module31_Out : ToWorkspace  VariableName=p_v_Module31  SaveFormat=Structure With Time  SampleTime=-1
  p_v_Module32_Out : ToWorkspace  VariableName=p_v_Module32  SaveFormat=Structure With Time  SampleTime=-1
  p_v_Module3_Out : ToWorkspace  VariableName=p_v_Module3  SaveFormat=Structure With Time  SampleTime=-1
  p_v_Module4_Out : ToWorkspace  VariableName=p_v_Module4  SaveFormat=Structure With Time  SampleTime=-1
  p_v_Module5_Out : ToWorkspace  VariableName=p_v_Module5  SaveFormat=Structure With Time  SampleTime=-1
  p_v_Module6_Out : ToWorkspace  VariableName=p_v_Module6  SaveFormat=Structure With Time  SampleTime=-1
  p_v_Module7_Out : ToWorkspace  VariableName=p_v_Module7  SaveFormat=Structure With Time  SampleTime=-1
  p_v_Module8_Out : ToWorkspace  VariableName=p_v_Module8  SaveFormat=Structure With Time  SampleTime=-1
  p_v_Module9_Out : ToWorkspace  VariableName=p_v_Module9  SaveFormat=Structure With Time  SampleTime=-1
  socCell_Module10_Out : ToWorkspace  VariableName=socCell_Module10  SaveFormat=Structure With Time  SampleTime=-1
  socCell_Module11_Out : ToWorkspace  VariableName=socCell_Module11  SaveFormat=Structure With Time  SampleTime=-1
  socCell_Module12_Out : ToWorkspace  VariableName=socCell_Module12  SaveFormat=Structure With Time  SampleTime=-1
  socCell_Module13_Out : ToWorkspace  VariableName=socCell_Module13  SaveFormat=Structure With Time  SampleTime=-1
  socCell_Module14_Out : ToWorkspace  VariableName=socCell_Module14  SaveFormat=Structure With Time  SampleTime=-1
  socCell_Module15_Out : ToWorkspace  VariableName=socCell_Module15  SaveFormat=Structure With Time  SampleTime=-1
  socCell_Module16_Out : ToWorkspace  VariableName=socCell_Module16  SaveFormat=Structure With Time  SampleTime=-1
  socCell_Module17_Out : ToWorkspace  VariableName=socCell_Module17  SaveFormat=Structure With Time  SampleTime=-1
  socCell_Module18_Out : ToWorkspace  VariableName=socCell_Module18  SaveFormat=Structure With Time  SampleTime=-1
  socCell_Module19_Out : ToWorkspace  VariableName=socCell_Module19  SaveFormat=Structure With Time  SampleTime=-1
  socCell_Module1_Out : ToWorkspace  VariableName=socCell_Module1  SaveFormat=Structure With Time  SampleTime=-1
  socCell_Module20_Out : ToWorkspace  VariableName=socCell_Module20  SaveFormat=Structure With Time  SampleTime=-1
  socCell_Module21_Out : ToWorkspace  VariableName=socCell_Module21  SaveFormat=Structure With Time  SampleTime=-1
  socCell_Module22_Out : ToWorkspace  VariableName=socCell_Module22  SaveFormat=Structure With Time  SampleTime=-1
  socCell_Module23_Out : ToWorkspace  VariableName=socCell_Module23  SaveFormat=Structure With Time  SampleTime=-1
  socCell_Module24_Out : ToWorkspace  VariableName=socCell_Module24  SaveFormat=Structure With Time  SampleTime=-1
  socCell_Module25_Out : ToWorkspace  VariableName=socCell_Module25  SaveFormat=Structure With Time  SampleTime=-1
  socCell_Module26_Out : ToWorkspace  VariableName=socCell_Module26  SaveFormat=Structure With Time  SampleTime=-1
  socCell_Module27_Out : ToWorkspace  VariableName=socCell_Module27  SaveFormat=Structure With Time  SampleTime=-1
  socCell_Module28_Out : ToWorkspace  VariableName=socCell_Module28  SaveFormat=Structure With Time  SampleTime=-1
  socCell_Module29_Out : ToWorkspace  VariableName=socCell_Module29  SaveFormat=Structure With Time  SampleTime=-1
  socCell_Module2_Out : ToWorkspace  VariableName=socCell_Module2  SaveFormat=Structure With Time  SampleTime=-1
  socCell_Module30_Out : ToWorkspace  VariableName=socCell_Module30  SaveFormat=Structure With Time  SampleTime=-1
  socCell_Module31_Out : ToWorkspace  VariableName=socCell_Module31  SaveFormat=Structure With Time  SampleTime=-1
  socCell_Module32_Out : ToWorkspace  VariableName=socCell_Module32  SaveFormat=Structure With Time  SampleTime=-1
  socCell_Module3_Out : ToWorkspace  VariableName=socCell_Module3  SaveFormat=Structure With Time  SampleTime=-1
  socCell_Module4_Out : ToWorkspace  VariableName=socCell_Module4  SaveFormat=Structure With Time  SampleTime=-1
  socCell_Module5_Out : ToWorkspace  VariableName=socCell_Module5  SaveFormat=Structure With Time  SampleTime=-1
  socCell_Module6_Out : ToWorkspace  VariableName=socCell_Module6  SaveFormat=Structure With Time  SampleTime=-1
  socCell_Module7_Out : ToWorkspace  VariableName=socCell_Module7  SaveFormat=Structure With Time  SampleTime=-1
  socCell_Module8_Out : ToWorkspace  VariableName=socCell_Module8  SaveFormat=Structure With Time  SampleTime=-1
  socCell_Module9_Out : ToWorkspace  VariableName=socCell_Module9  SaveFormat=Structure With Time  SampleTime=-1
  socParallelAssembly_Module10_Out : ToWorkspace  VariableName=socParallelAssembly_Module10  SaveFormat=Structure With Time  SampleTime=-1
  socParallelAssembly_Module11_Out : ToWorkspace  VariableName=socParallelAssembly_Module11  SaveFormat=Structure With Time  SampleTime=-1
  socParallelAssembly_Module12_Out : ToWorkspace  VariableName=socParallelAssembly_Module12  SaveFormat=Structure With Time  SampleTime=-1
  socParallelAssembly_Module13_Out : ToWorkspace  VariableName=socParallelAssembly_Module13  SaveFormat=Structure With Time  SampleTime=-1
  socParallelAssembly_Module14_Out : ToWorkspace  VariableName=socParallelAssembly_Module14  SaveFormat=Structure With Time  SampleTime=-1
  socParallelAssembly_Module15_Out : ToWorkspace  VariableName=socParallelAssembly_Module15  SaveFormat=Structure With Time  SampleTime=-1
  socParallelAssembly_Module16_Out : ToWorkspace  VariableName=socParallelAssembly_Module16  SaveFormat=Structure With Time  SampleTime=-1
  socParallelAssembly_Module17_Out : ToWorkspace  VariableName=socParallelAssembly_Module17  SaveFormat=Structure With Time  SampleTime=-1
  socParallelAssembly_Module18_Out : ToWorkspace  VariableName=socParallelAssembly_Module18  SaveFormat=Structure With Time  SampleTime=-1
  socParallelAssembly_Module19_Out : ToWorkspace  VariableName=socParallelAssembly_Module19  SaveFormat=Structure With Time  SampleTime=-1
  socParallelAssembly_Module1_Out : ToWorkspace  VariableName=socParallelAssembly_Module1  SaveFormat=Structure With Time  SampleTime=-1
  socParallelAssembly_Module20_Out : ToWorkspace  VariableName=socParallelAssembly_Module20  SaveFormat=Structure With Time  SampleTime=-1
  socParallelAssembly_Module21_Out : ToWorkspace  VariableName=socParallelAssembly_Module21  SaveFormat=Structure With Time  SampleTime=-1
  socParallelAssembly_Module22_Out : ToWorkspace  VariableName=socParallelAssembly_Module22  SaveFormat=Structure With Time  SampleTime=-1
  socParallelAssembly_Module23_Out : ToWorkspace  VariableName=socParallelAssembly_Module23  SaveFormat=Structure With Time  SampleTime=-1
  socParallelAssembly_Module24_Out : ToWorkspace  VariableName=socParallelAssembly_Module24  SaveFormat=Structure With Time  SampleTime=-1
  socParallelAssembly_Module25_Out : ToWorkspace  VariableName=socParallelAssembly_Module25  SaveFormat=Structure With Time  SampleTime=-1
  socParallelAssembly_Module26_Out : ToWorkspace  VariableName=socParallelAssembly_Module26  SaveFormat=Structure With Time  SampleTime=-1
  socParallelAssembly_Module27_Out : ToWorkspace  VariableName=socParallelAssembly_Module27  SaveFormat=Structure With Time  SampleTime=-1
  socParallelAssembly_Module28_Out : ToWorkspace  VariableName=socParallelAssembly_Module28  SaveFormat=Structure With Time  SampleTime=-1
  socParallelAssembly_Module29_Out : ToWorkspace  VariableName=socParallelAssembly_Module29  SaveFormat=Structure With Time  SampleTime=-1
  socParallelAssembly_Module2_Out : ToWorkspace  VariableName=socParallelAssembly_Module2  SaveFormat=Structure With Time  SampleTime=-1
  socParallelAssembly_Module30_Out : ToWorkspace  VariableName=socParallelAssembly_Module30  SaveFormat=Structure With Time  SampleTime=-1
  socParallelAssembly_Module31_Out : ToWorkspace  VariableName=socParallelAssembly_Module31  SaveFormat=Structure With Time  SampleTime=-1
  socParallelAssembly_Module32_Out : ToWorkspace  VariableName=socParallelAssembly_Module32  SaveFormat=Structure With Time  SampleTime=-1
  socParallelAssembly_Module3_Out : ToWorkspace  VariableName=socParallelAssembly_Module3  SaveFormat=Structure With Time  SampleTime=-1
  socParallelAssembly_Module4_Out : ToWorkspace  VariableName=socParallelAssembly_Module4  SaveFormat=Structure With Time  SampleTime=-1
  socParallelAssembly_Module5_Out : ToWorkspace  VariableName=socParallelAssembly_Module5  SaveFormat=Structure With Time  SampleTime=-1
  socParallelAssembly_Module6_Out : ToWorkspace  VariableName=socParallelAssembly_Module6  SaveFormat=Structure With Time  SampleTime=-1
  socParallelAssembly_Module7_Out : ToWorkspace  VariableName=socParallelAssembly_Module7  SaveFormat=Structure With Time  SampleTime=-1
  socParallelAssembly_Module8_Out : ToWorkspace  VariableName=socParallelAssembly_Module8  SaveFormat=Structure With Time  SampleTime=-1
  socParallelAssembly_Module9_Out : ToWorkspace  VariableName=socParallelAssembly_Module9  SaveFormat=Structure With Time  SampleTime=-1
  vParallelAssembly_Module10_Out : ToWorkspace  VariableName=vParallelAssembly_Module10  SaveFormat=Structure With Time  SampleTime=-1
  vParallelAssembly_Module11_Out : ToWorkspace  VariableName=vParallelAssembly_Module11  SaveFormat=Structure With Time  SampleTime=-1
  vParallelAssembly_Module12_Out : ToWorkspace  VariableName=vParallelAssembly_Module12  SaveFormat=Structure With Time  SampleTime=-1
  vParallelAssembly_Module13_Out : ToWorkspace  VariableName=vParallelAssembly_Module13  SaveFormat=Structure With Time  SampleTime=-1
  vParallelAssembly_Module14_Out : ToWorkspace  VariableName=vParallelAssembly_Module14  SaveFormat=Structure With Time  SampleTime=-1
  vParallelAssembly_Module15_Out : ToWorkspace  VariableName=vParallelAssembly_Module15  SaveFormat=Structure With Time  SampleTime=-1
  vParallelAssembly_Module16_Out : ToWorkspace  VariableName=vParallelAssembly_Module16  SaveFormat=Structure With Time  SampleTime=-1
  vParallelAssembly_Module17_Out : ToWorkspace  VariableName=vParallelAssembly_Module17  SaveFormat=Structure With Time  SampleTime=-1
  vParallelAssembly_Module18_Out : ToWorkspace  VariableName=vParallelAssembly_Module18  SaveFormat=Structure With Time  SampleTime=-1
  vParallelAssembly_Module19_Out : ToWorkspace  VariableName=vParallelAssembly_Module19  SaveFormat=Structure With Time  SampleTime=-1
  vParallelAssembly_Module1_Out : ToWorkspace  VariableName=vParallelAssembly_Module1  SaveFormat=Structure With Time  SampleTime=-1
  vParallelAssembly_Module20_Out : ToWorkspace  VariableName=vParallelAssembly_Module20  SaveFormat=Structure With Time  SampleTime=-1
  vParallelAssembly_Module21_Out : ToWorkspace  VariableName=vParallelAssembly_Module21  SaveFormat=Structure With Time  SampleTime=-1
  vParallelAssembly_Module22_Out : ToWorkspace  VariableName=vParallelAssembly_Module22  SaveFormat=Structure With Time  SampleTime=-1
  vParallelAssembly_Module23_Out : ToWorkspace  VariableName=vParallelAssembly_Module23  SaveFormat=Structure With Time  SampleTime=-1
  vParallelAssembly_Module24_Out : ToWorkspace  VariableName=vParallelAssembly_Module24  SaveFormat=Structure With Time  SampleTime=-1
  vParallelAssembly_Module25_Out : ToWorkspace  VariableName=vParallelAssembly_Module25  SaveFormat=Structure With Time  SampleTime=-1
  vParallelAssembly_Module26_Out : ToWorkspace  VariableName=vParallelAssembly_Module26  SaveFormat=Structure With Time  SampleTime=-1
  vParallelAssembly_Module27_Out : ToWorkspace  VariableName=vParallelAssembly_Module27  SaveFormat=Structure With Time  SampleTime=-1
  vParallelAssembly_Module28_Out : ToWorkspace  VariableName=vParallelAssembly_Module28  SaveFormat=Structure With Time  SampleTime=-1
  vParallelAssembly_Module29_Out : ToWorkspace  VariableName=vParallelAssembly_Module29  SaveFormat=Structure With Time  SampleTime=-1
  vParallelAssembly_Module2_Out : ToWorkspace  VariableName=vParallelAssembly_Module2  SaveFormat=Structure With Time  SampleTime=-1
  vParallelAssembly_Module30_Out : ToWorkspace  VariableName=vParallelAssembly_Module30  SaveFormat=Structure With Time  SampleTime=-1
  vParallelAssembly_Module31_Out : ToWorkspace  VariableName=vParallelAssembly_Module31  SaveFormat=Structure With Time  SampleTime=-1
  vParallelAssembly_Module32_Out : ToWorkspace  VariableName=vParallelAssembly_Module32  SaveFormat=Structure With Time  SampleTime=-1
  vParallelAssembly_Module3_Out : ToWorkspace  VariableName=vParallelAssembly_Module3  SaveFormat=Structure With Time  SampleTime=-1
  vParallelAssembly_Module4_Out : ToWorkspace  VariableName=vParallelAssembly_Module4  SaveFormat=Structure With Time  SampleTime=-1
  vParallelAssembly_Module5_Out : ToWorkspace  VariableName=vParallelAssembly_Module5  SaveFormat=Structure With Time  SampleTime=-1
  vParallelAssembly_Module6_Out : ToWorkspace  VariableName=vParallelAssembly_Module6  SaveFormat=Structure With Time  SampleTime=-1
  vParallelAssembly_Module7_Out : ToWorkspace  VariableName=vParallelAssembly_Module7  SaveFormat=Structure With Time  SampleTime=-1
  vParallelAssembly_Module8_Out : ToWorkspace  VariableName=vParallelAssembly_Module8  SaveFormat=Structure With Time  SampleTime=-1
  vParallelAssembly_Module9_Out : ToWorkspace  VariableName=vParallelAssembly_Module9  SaveFormat=Structure With Time  SampleTime=-1
  Out1 : Outport
  wires:
  In1/1 -> Out1/1
  Probe_Module1/1 -> AmbH_T_Module1_Out/1
  Probe_Module1/2 -> batteryCurrent_Module1_Out/1
  Probe_Module1/3 -> batteryTemperature_Module1_Out/1
  Probe_Module1/4 -> batteryVoltage_Module1_Out/1
  Probe_Module1/5 -> n_v_Module1_Out/1
  Probe_Module1/6 -> numCycles_Module1_Out/1
  Probe_Module1/7 -> p_v_Module1_Out/1
  Probe_Module1/8 -> socCell_Module1_Out/1
  Probe_Module1/9 -> socParallelAssembly_Module1_Out/1
  Probe_Module1/10 -> vParallelAssembly_Module1_Out/1
  Probe_Module2/1 -> AmbH_T_Module2_Out/1
  Probe_Module2/2 -> batteryCurrent_Module2_Out/1
  Probe_Module2/3 -> batteryTemperature_Module2_Out/1
  Probe_Module2/4 -> batteryVoltage_Module2_Out/1
  Probe_Module2/5 -> n_v_Module2_Out/1
  Probe_Module2/6 -> numCycles_Module2_Out/1
  Probe_Module2/7 -> p_v_Module2_Out/1
  Probe_Module2/8 -> socCell_Module2_Out/1
  Probe_Module2/9 -> socParallelAssembly_Module2_Out/1
  Probe_Module2/10 -> vParallelAssembly_Module2_Out/1
  Probe_Module3/1 -> AmbH_T_Module3_Out/1
  Probe_Module3/2 -> batteryCurrent_Module3_Out/1
  Probe_Module3/3 -> batteryTemperature_Module3_Out/1
  Probe_Module3/4 -> batteryVoltage_Module3_Out/1
  Probe_Module3/5 -> n_v_Module3_Out/1
  Probe_Module3/6 -> numCycles_Module3_Out/1
  Probe_Module3/7 -> p_v_Module3_Out/1
  Probe_Module3/8 -> socCell_Module3_Out/1
  Probe_Module3/9 -> socParallelAssembly_Module3_Out/1
  Probe_Module3/10 -> vParallelAssembly_Module3_Out/1
  Probe_Module4/1 -> AmbH_T_Module4_Out/1
  Probe_Module4/2 -> batteryCurrent_Module4_Out/1
  Probe_Module4/3 -> batteryTemperature_Module4_Out/1
  Probe_Module4/4 -> batteryVoltage_Module4_Out/1
  Probe_Module4/5 -> n_v_Module4_Out/1
  Probe_Module4/6 -> numCycles_Module4_Out/1
  Probe_Module4/7 -> p_v_Module4_Out/1
  Probe_Module4/8 -> socCell_Module4_Out/1
  Probe_Module4/9 -> socParallelAssembly_Module4_Out/1
  Probe_Module4/10 -> vParallelAssembly_Module4_Out/1
  Probe_Module5/1 -> AmbH_T_Module5_Out/1
  Probe_Module5/2 -> batteryCurrent_Module5_Out/1
  Probe_Module5/3 -> batteryTemperature_Module5_Out/1
  Probe_Module5/4 -> batteryVoltage_Module5_Out/1
  Probe_Module5/5 -> n_v_Module5_Out/1
  Probe_Module5/6 -> numCycles_Module5_Out/1
  Probe_Module5/7 -> p_v_Module5_Out/1
  Probe_Module5/8 -> socCell_Module5_Out/1
  Probe_Module5/9 -> socParallelAssembly_Module5_Out/1
  Probe_Module5/10 -> vParallelAssembly_Module5_Out/1
  Probe_Module6/1 -> AmbH_T_Module6_Out/1
  Probe_Module6/2 -> batteryCurrent_Module6_Out/1
  Probe_Module6/3 -> batteryTemperature_Module6_Out/1
  Probe_Module6/4 -> batteryVoltage_Module6_Out/1
  Probe_Module6/5 -> n_v_Module6_Out/1
  Probe_Module6/6 -> numCycles_Module6_Out/1
  Probe_Module6/7 -> p_v_Module6_Out/1
  Probe_Module6/8 -> socCell_Module6_Out/1
  Probe_Module6/9 -> socParallelAssembly_Module6_Out/1
  Probe_Module6/10 -> vParallelAssembly_Module6_Out/1
  Probe_Module7/1 -> AmbH_T_Module7_Out/1
  Probe_Module7/2 -> batteryCurrent_Module7_Out/1
  Probe_Module7/3 -> batteryTemperature_Module7_Out/1
  Probe_Module7/4 -> batteryVoltage_Module7_Out/1
  Probe_Module7/5 -> n_v_Module7_Out/1
  Probe_Module7/6 -> numCycles_Module7_Out/1
  Probe_Module7/7 -> p_v_Module7_Out/1
  Probe_Module7/8 -> socCell_Module7_Out/1
  Probe_Module7/9 -> socParallelAssembly_Module7_Out/1
  Probe_Module7/10 -> vParallelAssembly_Module7_Out/1
  Probe_Module8/1 -> AmbH_T_Module8_Out/1
  Probe_Module8/2 -> batteryCurrent_Module8_Out/1
  Probe_Module8/3 -> batteryTemperature_Module8_Out/1
  Probe_Module8/4 -> batteryVoltage_Module8_Out/1
  Probe_Module8/5 -> n_v_Module8_Out/1
  Probe_Module8/6 -> numCycles_Module8_Out/1
  Probe_Module8/7 -> p_v_Module8_Out/1
  Probe_Module8/8 -> socCell_Module8_Out/1
  Probe_Module8/9 -> socParallelAssembly_Module8_Out/1
  Probe_Module8/10 -> vParallelAssembly_Module8_Out/1
  Probe_Module9/1 -> AmbH_T_Module9_Out/1
  Probe_Module9/2 -> batteryCurrent_Module9_Out/1
  Probe_Module9/3 -> batteryTemperature_Module9_Out/1
  Probe_Module9/4 -> batteryVoltage_Module9_Out/1
  Probe_Module9/5 -> n_v_Module9_Out/1
  Probe_Module9/6 -> numCycles_Module9_Out/1
  Probe_Module9/7 -> p_v_Module9_Out/1
  Probe_Module9/8 -> socCell_Module9_Out/1
  Probe_Module9/9 -> socParallelAssembly_Module9_Out/1
  Probe_Module9/10 -> vParallelAssembly_Module9_Out/1
  Probe_Module10/1 -> AmbH_T_Module10_Out/1
  Probe_Module10/2 -> batteryCurrent_Module10_Out/1
  Probe_Module10/3 -> batteryTemperature_Module10_Out/1
  Probe_Module10/4 -> batteryVoltage_Module10_Out/1
  Probe_Module10/5 -> n_v_Module10_Out/1
  Probe_Module10/6 -> numCycles_Module10_Out/1
  Probe_Module10/7 -> p_v_Module10_Out/1
  Probe_Module10/8 -> socCell_Module10_Out/1
  Probe_Module10/9 -> socParallelAssembly_Module10_Out/1
  Probe_Module10/10 -> vParallelAssembly_Module10_Out/1
  Probe_Module11/1 -> AmbH_T_Module11_Out/1
  Probe_Module11/2 -> batteryCurrent_Module11_Out/1
  Probe_Module11/3 -> batteryTemperature_Module11_Out/1
  Probe_Module11/4 -> batteryVoltage_Module11_Out/1
  Probe_Module11/5 -> n_v_Module11_Out/1
  Probe_Module11/6 -> numCycles_Module11_Out/1
  Probe_Module11/7 -> p_v_Module11_Out/1
  Probe_Module11/8 -> socCell_Module11_Out/1
  Probe_Module11/9 -> socParallelAssembly_Module11_Out/1
  Probe_Module11/10 -> vParallelAssembly_Module11_Out/1
  Probe_Module12/1 -> AmbH_T_Module12_Out/1
  Probe_Module12/2 -> batteryCurrent_Module12_Out/1
  Probe_Module12/3 -> batteryTemperature_Module12_Out/1
  Probe_Module12/4 -> batteryVoltage_Module12_Out/1
  Probe_Module12/5 -> n_v_Module12_Out/1
  Probe_Module12/6 -> numCycles_Module12_Out/1
  Probe_Module12/7 -> p_v_Module12_Out/1
  Probe_Module12/8 -> socCell_Module12_Out/1
  Probe_Module12/9 -> socParallelAssembly_Module12_Out/1
  Probe_Module12/10 -> vParallelAssembly_Module12_Out/1
  Probe_Module13/1 -> AmbH_T_Module13_Out/1
  Probe_Module13/2 -> batteryCurrent_Module13_Out/1
  Probe_Module13/3 -> batteryTemperature_Module13_Out/1
  Probe_Module13/4 -> batteryVoltage_Module13_Out/1
  Probe_Module13/5 -> n_v_Module13_Out/1
  Probe_Module13/6 -> numCycles_Module13_Out/1
  Probe_Module13/7 -> p_v_Module13_Out/1
  Probe_Module13/8 -> socCell_Module13_Out/1
  Probe_Module13/9 -> socParallelAssembly_Module13_Out/1
  Probe_Module13/10 -> vParallelAssembly_Module13_Out/1
  Probe_Module14/1 -> AmbH_T_Module14_Out/1
  Probe_Module14/2 -> batteryCurrent_Module14_Out/1
  Probe_Module14/3 -> batteryTemperature_Module14_Out/1
  Probe_Module14/4 -> batteryVoltage_Module14_Out/1
  Probe_Module14/5 -> n_v_Module14_Out/1
  Probe_Module14/6 -> numCycles_Module14_Out/1
  Probe_Module14/7 -> p_v_Module14_Out/1
  Probe_Module14/8 -> socCell_Module14_Out/1
  Probe_Module14/9 -> socParallelAssembly_Module14_Out/1
  Probe_Module14/10 -> vParallelAssembly_Module14_Out/1
  Probe_Module15/1 -> AmbH_T_Module15_Out/1
  Probe_Module15/2 -> batteryCurrent_Module15_Out/1
  Probe_Module15/3 -> batteryTemperature_Module15_Out/1
  Probe_Module15/4 -> batteryVoltage_Module15_Out/1
  Probe_Module15/5 -> n_v_Module15_Out/1
  Probe_Module15/6 -> numCycles_Module15_Out/1
  Probe_Module15/7 -> p_v_Module15_Out/1
  Probe_Module15/8 -> socCell_Module15_Out/1
  Probe_Module15/9 -> socParallelAssembly_Module15_Out/1
  Probe_Module15/10 -> vParallelAssembly_Module15_Out/1
  Probe_Module16/1 -> AmbH_T_Module16_Out/1
  Probe_Module16/2 -> batteryCurrent_Module16_Out/1
  Probe_Module16/3 -> batteryTemperature_Module16_Out/1
  Probe_Module16/4 -> batteryVoltage_Module16_Out/1
  Probe_Module16/5 -> n_v_Module16_Out/1
  Probe_Module16/6 -> numCycles_Module16_Out/1
  Probe_Module16/7 -> p_v_Module16_Out/1
  Probe_Module16/8 -> socCell_Module16_Out/1
  Probe_Module16/9 -> socParallelAssembly_Module16_Out/1
  Probe_Module16/10 -> vParallelAssembly_Module16_Out/1
  Probe_Module17/1 -> AmbH_T_Module17_Out/1
  Probe_Module17/2 -> batteryCurrent_Module17_Out/1
  Probe_Module17/3 -> batteryTemperature_Module17_Out/1
  Probe_Module17/4 -> batteryVoltage_Module17_Out/1
  Probe_Module17/5 -> n_v_Module17_Out/1
  Probe_Module17/6 -> numCycles_Module17_Out/1
  Probe_Module17/7 -> p_v_Module17_Out/1
  Probe_Module17/8 -> socCell_Module17_Out/1
  Probe_Module17/9 -> socParallelAssembly_Module17_Out/1
  Probe_Module17/10 -> vParallelAssembly_Module17_Out/1
  Probe_Module18/1 -> AmbH_T_Module18_Out/1
  Probe_Module18/2 -> batteryCurrent_Module18_Out/1
  Probe_Module18/3 -> batteryTemperature_Module18_Out/1
  Probe_Module18/4 -> batteryVoltage_Module18_Out/1
  Probe_Module18/5 -> n_v_Module18_Out/1
  Probe_Module18/6 -> numCycles_Module18_Out/1
  Probe_Module18/7 -> p_v_Module18_Out/1
  Probe_Module18/8 -> socCell_Module18_Out/1
  Probe_Module18/9 -> socParallelAssembly_Module18_Out/1
  Probe_Module18/10 -> vParallelAssembly_Module18_Out/1
  Probe_Module19/1 -> AmbH_T_Module19_Out/1
  Probe_Module19/2 -> batteryCurrent_Module19_Out/1
  Probe_Module19/3 -> batteryTemperature_Module19_Out/1
  Probe_Module19/4 -> batteryVoltage_Module19_Out/1
  Probe_Module19/5 -> n_v_Module19_Out/1
  Probe_Module19/6 -> numCycles_Module19_Out/1
  Probe_Module19/7 -> p_v_Module19_Out/1
  Probe_Module19/8 -> socCell_Module19_Out/1
  Probe_Module19/9 -> socParallelAssembly_Module19_Out/1
  Probe_Module19/10 -> vParallelAssembly_Module19_Out/1
  Probe_Module20/1 -> AmbH_T_Module20_Out/1
  Probe_Module20/2 -> batteryCurrent_Module20_Out/1
  Probe_Module20/3 -> batteryTemperature_Module20_Out/1
  Probe_Module20/4 -> batteryVoltage_Module20_Out/1
  Probe_Module20/5 -> n_v_Module20_Out/1
  Probe_Module20/6 -> numCycles_Module20_Out/1
  Probe_Module20/7 -> p_v_Module20_Out/1
  Probe_Module20/8 -> socCell_Module20_Out/1
  Probe_Module20/9 -> socParallelAssembly_Module20_Out/1
  Probe_Module20/10 -> vParallelAssembly_Module20_Out/1
  Probe_Module21/1 -> AmbH_T_Module21_Out/1
  Probe_Module21/2 -> batteryCurrent_Module21_Out/1
  Probe_Module21/3 -> batteryTemperature_Module21_Out/1
  Probe_Module21/4 -> batteryVoltage_Module21_Out/1
  Probe_Module21/5 -> n_v_Module21_Out/1
  Probe_Module21/6 -> numCycles_Module21_Out/1
  Probe_Module21/7 -> p_v_Module21_Out/1
  Probe_Module21/8 -> socCell_Module21_Out/1
  Probe_Module21/9 -> socParallelAssembly_Module21_Out/1
  Probe_Module21/10 -> vParallelAssembly_Module21_Out/1
  Probe_Module22/1 -> AmbH_T_Module22_Out/1
  Probe_Module22/2 -> batteryCurrent_Module22_Out/1
  Probe_Module22/3 -> batteryTemperature_Module22_Out/1
  Probe_Module22/4 -> batteryVoltage_Module22_Out/1
  Probe_Module22/5 -> n_v_Module22_Out/1
  Probe_Module22/6 -> numCycles_Module22_Out/1
  Probe_Module22/7 -> p_v_Module22_Out/1
  Probe_Module22/8 -> socCell_Module22_Out/1
  Probe_Module22/9 -> socParallelAssembly_Module22_Out/1
  Probe_Module22/10 -> vParallelAssembly_Module22_Out/1
  Probe_Module23/1 -> AmbH_T_Module23_Out/1
  Probe_Module23/2 -> batteryCurrent_Module23_Out/1
  Probe_Module23/3 -> batteryTemperature_Module23_Out/1
  Probe_Module23/4 -> batteryVoltage_Module23_Out/1
  Probe_Module23/5 -> n_v_Module23_Out/1
  Probe_Module23/6 -> numCycles_Module23_Out/1
  Probe_Module23/7 -> p_v_Module23_Out/1
  Probe_Module23/8 -> socCell_Module23_Out/1
  Probe_Module23/9 -> socParallelAssembly_Module23_Out/1
  Probe_Module23/10 -> vParallelAssembly_Module23_Out/1
  Probe_Module24/1 -> AmbH_T_Module24_Out/1
  Probe_Module24/2 -> batteryCurrent_Module24_Out/1
  Probe_Module24/3 -> batteryTemperature_Module24_Out/1
  Probe_Module24/4 -> batteryVoltage_Module24_Out/1
  Probe_Module24/5 -> n_v_Module24_Out/1
  Probe_Module24/6 -> numCycles_Module24_Out/1
  Probe_Module24/7 -> p_v_Module24_Out/1
  Probe_Module24/8 -> socCell_Module24_Out/1
  Probe_Module24/9 -> socParallelAssembly_Module24_Out/1
  Probe_Module24/10 -> vParallelAssembly_Module24_Out/1
  Probe_Module25/1 -> AmbH_T_Module25_Out/1
  Probe_Module25/2 -> batteryCurrent_Module25_Out/1
  Probe_Module25/3 -> batteryTemperature_Module25_Out/1
  Probe_Module25/4 -> batteryVoltage_Module25_Out/1
  Probe_Module25/5 -> n_v_Module25_Out/1
  Probe_Module25/6 -> numCycles_Module25_Out/1
  Probe_Module25/7 -> p_v_Module25_Out/1
  Probe_Module25/8 -> socCell_Module25_Out/1
  Probe_Module25/9 -> socParallelAssembly_Module25_Out/1
  Probe_Module25/10 -> vParallelAssembly_Module25_Out/1
  Probe_Module26/1 -> AmbH_T_Module26_Out/1
  Probe_Module26/2 -> batteryCurrent_Module26_Out/1
  Probe_Module26/3 -> batteryTemperature_Module26_Out/1
  Probe_Module26/4 -> batteryVoltage_Module26_Out/1
  Probe_Module26/5 -> n_v_Module26_Out/1
  Probe_Module26/6 -> numCycles_Module26_Out/1
  Probe_Module26/7 -> p_v_Module26_Out/1
  Probe_Module26/8 -> socCell_Module26_Out/1
  Probe_Module26/9 -> socParallelAssembly_Module26_Out/1
  Probe_Module26/10 -> vParallelAssembly_Module26_Out/1
  Probe_Module27/1 -> AmbH_T_Module27_Out/1
  Probe_Module27/2 -> batteryCurrent_Module27_Out/1
  Probe_Module27/3 -> batteryTemperature_Module27_Out/1
  Probe_Module27/4 -> batteryVoltage_Module27_Out/1
  Probe_Module27/5 -> n_v_Module27_Out/1
  Probe_Module27/6 -> numCycles_Module27_Out/1
  Probe_Module27/7 -> p_v_Module27_Out/1
  Probe_Module27/8 -> socCell_Module27_Out/1
  Probe_Module27/9 -> socParallelAssembly_Module27_Out/1
  Probe_Module27/10 -> vParallelAssembly_Module27_Out/1
  Probe_Module28/1 -> AmbH_T_Module28_Out/1
  Probe_Module28/2 -> batteryCurrent_Module28_Out/1
  Probe_Module28/3 -> batteryTemperature_Module28_Out/1
  Probe_Module28/4 -> batteryVoltage_Module28_Out/1
  Probe_Module28/5 -> n_v_Module28_Out/1
  Probe_Module28/6 -> numCycles_Module28_Out/1
  Probe_Module28/7 -> p_v_Module28_Out/1
  Probe_Module28/8 -> socCell_Module28_Out/1
  Probe_Module28/9 -> socParallelAssembly_Module28_Out/1
  Probe_Module28/10 -> vParallelAssembly_Module28_Out/1
  Probe_Module29/1 -> AmbH_T_Module29_Out/1
  Probe_Module29/2 -> batteryCurrent_Module29_Out/1
  Probe_Module29/3 -> batteryTemperature_Module29_Out/1
  Probe_Module29/4 -> batteryVoltage_Module29_Out/1
  Probe_Module29/5 -> n_v_Module29_Out/1
  Probe_Module29/6 -> numCycles_Module29_Out/1
  Probe_Module29/7 -> p_v_Module29_Out/1
  Probe_Module29/8 -> socCell_Module29_Out/1
  Probe_Module29/9 -> socParallelAssembly_Module29_Out/1
  Probe_Module29/10 -> vParallelAssembly_Module29_Out/1
  Probe_Module30/1 -> AmbH_T_Module30_Out/1
  Probe_Module30/2 -> batteryCurrent_Module30_Out/1
  Probe_Module30/3 -> batteryTemperature_Module30_Out/1
  Probe_Module30/4 -> batteryVoltage_Module30_Out/1
  Probe_Module30/5 -> n_v_Module30_Out/1
  Probe_Module30/6 -> numCycles_Module30_Out/1
  Probe_Module30/7 -> p_v_Module30_Out/1
  Probe_Module30/8 -> socCell_Module30_Out/1
  Probe_Module30/9 -> socParallelAssembly_Module30_Out/1
  Probe_Module30/10 -> vParallelAssembly_Module30_Out/1
  Probe_Module31/1 -> AmbH_T_Module31_Out/1
  Probe_Module31/2 -> batteryCurrent_Module31_Out/1
  Probe_Module31/3 -> batteryTemperature_Module31_Out/1
  Probe_Module31/4 -> batteryVoltage_Module31_Out/1
  Probe_Module31/5 -> n_v_Module31_Out/1
  Probe_Module31/6 -> numCycles_Module31_Out/1
  Probe_Module31/7 -> p_v_Module31_Out/1
  Probe_Module31/8 -> socCell_Module31_Out/1
  Probe_Module31/9 -> socParallelAssembly_Module31_Out/1
  Probe_Module31/10 -> vParallelAssembly_Module31_Out/1
  Probe_Module32/1 -> AmbH_T_Module32_Out/1
  Probe_Module32/2 -> batteryCurrent_Module32_Out/1
  Probe_Module32/3 -> batteryTemperature_Module32_Out/1
  Probe_Module32/4 -> batteryVoltage_Module32_Out/1
  Probe_Module32/5 -> n_v_Module32_Out/1
  Probe_Module32/6 -> numCycles_Module32_Out/1
  Probe_Module32/7 -> p_v_Module32_Out/1
  Probe_Module32/8 -> socCell_Module32_Out/1
  Probe_Module32/9 -> socParallelAssembly_Module32_Out/1
  Probe_Module32/10 -> vParallelAssembly_Module32_Out/1
